simulink model "code_gen_HeadingHold"  (Simulink 7.5)
settings: Solver=FixedStepDiscrete  SolverMode=SingleTasking  StartTime=0.0  StopTime=10.0  FixedStep=0.01  RelTol=1e-3
InitFcn:
  | boat_constants
values from neighbouring files (symbols this model uses):
  figure8_waypoints = int32([ ... (first row only)    [boat_constants.m]
  OC2max = 49999    [boat_constants.m]    (also in simulation_constants.m)
  sampling_waypoints = int32([ ... (first row only)    [boat_constants.m]
  T_step = 0.01    [boat_constants.m]    (also in common.m)
  test_waypoints = int32([ ... (first row only)    [boat_constants.m]
undefined symbols (not defined in the file or in its folder): clearGpsData, clearSensorData, cpInitCommunications, DataEEInitAndClear, DataEEWrite, DiscIntNeverNeededParam, ecan1_buffered_transmit_matlab, ecan1_error_status_matlab, ecan1_init, ecan1_receive_matlab, getGpsData, getSensorData, Init_onlyOnce, Init_Reset, initCalibrationRange, initGps, processNewCommData, processNewGpsData, setHilMode, u1, u2, uart1EnqueueStateData, uart2EnqueueActuatorData, y1
libraries: simulink x85, dsPICdrivers x44, uSimLib x6, simulink_need_slupdate x4, aerolibconvert2 x2
(part 3 of 6)

== system code_gen_HeadingHold/Sensor Inputs/Change UART Baudrate ==
  HIL : Inport
  Enable : EnablePort
  Data Type Conversion : DataTypeConversion  OutDataType=fixdt(1, 16)  OutScaling=2^0
  Reconfigure UART2 baud rate [commProtocol.c] : dsPICdrivers/OTHERS/C Function Call  Tag=dsPIC_dsPIC_CFunctionCall  FctUpdate=Output Function  fctName='setHilMode'  INPUT_SIZE=1  INPUT1=uint8  INPUT2=--  INPUT3=--  OUTPUT_SIZE=1  OUTPUT1=--  SampleTime=T_step  InputType=[ 2 ]  OutputType=[ ]  FctDeclaration=extern void setHilMode(uint8_T u1);  FctCall=setHilMode(%u1);  OrderingInOutPopup=None  FctStart=None  FctStart_Name=Init_onlyOnce  FctStart_Declaration=inline extern void Init_onlyOnce();  FctStart_Call=Init_onlyOnce();  FctInit=None  FctInit_Name=Init_Reset  FctInit_Declaration=inline extern void Init_Reset();  FctInit_Call=Init_Reset();  PinDigitalInput=[]  PinDigitalOutput=[]  AnalogueInput=[]
  wires:
  HIL/1 -> Data Type Conversion/1
  Data Type Conversion/1 -> Reconfigure UART2 baud rate [commProtocol.c]/1

== system code_gen_HeadingHold/Sensor Inputs/Estop detection ==
  note: The below ECAN1 RX block is for checking for status messages.
      | If a status message hasn't been received for 2.1 seconds, a reset
      | signal is activated. The status messages for the ACS300 are not
      | sent when it is in reset, so this will catch when the estop is active.
      |
      | This also serves to check that the CAN hardware is working correctly,
      | which I have had trouble with in the past.
  Compare To Constant : simulink/Logic and Bit Operations/Compare To Constant  SystemSampleTime=-1  relop===  const=1026  LogicOutDataTypeMode=boolean
  Compare To Constant1 : simulink/Logic and Bit Operations/Compare To Constant  SystemSampleTime=-1  relop===  const=1  LogicOutDataTypeMode=boolean
  Constant1 : Constant  OutDataTypeMode=uint8  OutDataType=fixdt(1, 16)  OutScaling=2^0  OutDataTypeStr=uint8
  Data Store Memory : DataStoreMemory  DataStoreName=v_rpm  ReadBeforeWriteMsg=warning  WriteAfterWriteMsg=warning  WriteAfterReadMsg=warning  DataType=int16  OutDataType=fixdt(1, 16)  OutScaling=2^0  OutDataTypeStr=int16
  Data Store Read : DataStoreRead  Priority=2  DataStoreName=v_rpm  SampleTime=T_step
  Discrete-Time Integrator : DiscreteIntegrator  IntegratorMethod=Accumulation: Forward Euler  gainval=1  ExternalReset=level  SampleTime=-1  OutDataType=fixdt(1, 16)  OutScaling=2^0  LimitOutput=on  UpperSaturationLimit=50  LowerSaturationLimit=0  ShowSaturationPort=on  ICPrevOutput=DiscIntNeverNeededParam  ICPrevScaledInput=DiscIntNeverNeededParam
  If Action Subsystem : Subsystem  Priority=1  TreatAsAtomicUnit=on
  If1 : If  IfExpression=u1 == 1026  ShowElse=off
  Logical Operator5 : Logic  AllPortsSameDT=off  OutDataTypeMode=boolean  LogicDataType=fixdt(0, 8)  OutDataTypeStr=boolean
  Receive ECAN1 Message : Subsystem  mask(ECAN 1 Reception Block){ecan1_receive_sample_time=.01}
      mask prompts: ecan1_receive_sample_time "Sampling time"
      mask help:
      | This block will receive CAN messages over the ECAN1 peripheral on the dsPIC33f.
      | Outputs:
      | identifier - uint32 containing SID and EID
      | data - Variable-sized array (between 0 and 8) of uint8s
      | remote - boolean value specifying if this is a remote transmit request
      mask Display: disp('ECAN1 RX');
  Terminator1 : Terminator
  Terminator2 : Terminator
  Terminator3 : Terminator
  reset_estop : Outport
  tag scope: v_rpm=global
  wires:
  Receive ECAN1 Message/1(identifier) -> Compare To Constant/1, If1/1
  Constant1/1 -> Discrete-Time Integrator/1
  Compare To Constant/1 -> Logical Operator5/1
  Receive ECAN1 Message/4(new) -> Logical Operator5/2
  Logical Operator5/1 -> Discrete-Time Integrator/2
  Receive ECAN1 Message/2(data) -> If Action Subsystem/1(data)
  Receive ECAN1 Message/3(remote) -> Terminator1/1
  Receive ECAN1 Message/5(size) -> Terminator2/1
  Discrete-Time Integrator/2 -> Compare To Constant1/1
  Discrete-Time Integrator/1 -> Terminator3/1
  Compare To Constant1/1 -> reset_estop/1
  If1/1 -> If Action Subsystem/Action
  Data Store Read/1 -> [v_rpm]

== system code_gen_HeadingHold/Sensor Inputs/GPS ==
  Enable : EnablePort
  Bus Creator : BusCreator  Inputs=15
  Data Type Conversion : DataTypeConversion  OutDataTypeMode=boolean  OutDataType=fixdt(1, 16)  OutScaling=2^0  OutDataTypeStr=boolean  RndMeth=Simplest
  GPS Reception Status (LED D9) : dsPICdrivers/Digital I//O/Digital Output Write  Tag=dsPIC_Digital_Output  Priority=5  PORT=A  Pin=[6]  Simultaneous=off  OrderingInOutPopup=None
  Logical Operator4 : Logic  AllPortsSameDT=off  OutDataTypeMode=boolean  LogicDataType=fixdt(0, 8)  OutDataTypeStr=boolean
  Parse out new data since the last timestep [gps.c] : dsPICdrivers/OTHERS/C Function Call  Tag=dsPIC_dsPIC_CFunctionCall  FctUpdate=Output Function  fctName='processNewGpsData'  INPUT_SIZE=1  INPUT1=--  INPUT2=--  INPUT3=--  OUTPUT_SIZE=1  OUTPUT1=--  SampleTime=T_step  InputType=[ ]  OutputType=[ ]  FctDeclaration=extern void processNewGpsData();  FctCall=processNewGpsData();  OrderingInOutPopup=Output  FctStart=None  FctStart_Name=Init_onlyOnce  FctStart_Declaration=inline extern void Init_onlyOnce();  FctStart_Call=Init_onlyOnce();  FctInit=None  FctInit_Name=Init_Reset  FctInit_Declaration=inline extern void Init_Reset();  FctInit_Call=Init_Reset();  PinDigitalInput=[]  PinDigitalOutput=[]  AnalogueInput=[]
  Retrieve last GPS data [gps.c] : dsPICdrivers/OTHERS/C Function Call  Tag=dsPIC_dsPIC_CFunctionCall  FctUpdate=Output Function  fctName='getGpsData'  INPUT_SIZE=1  INPUT1=--  INPUT2=--  INPUT3=--  OUTPUT_SIZE=33  OUTPUT1=uint8  SampleTime=T_step  InputType=[ ]  OutputType=[ 2 ]  FctDeclaration=extern void getGpsData(uint8_T* y1);  FctCall=getGpsData(*%y1);  OrderingInOutPopup=Input  FctStart=None  FctStart_Name=Init_onlyOnce  FctStart_Declaration=inline extern void Init_onlyOnce();  FctStart_Call=Init_onlyOnce();  FctInit=None  FctInit_Name=Init_Reset  FctInit_Declaration=inline extern void Init_Reset();  FctInit_Call=Init_Reset();  PinDigitalInput=[]  PinDigitalOutput=[]  AnalogueInput=[]
  Unpack sensor data : Stateflow chart  TreatAsAtomicUnit=on
  GPS : Outport
  wires:
  Bus Creator/1 -> GPS/1
  Parse out new data since the last timestep [gps.c]/1 -> Retrieve last GPS data [gps.c]/1
  Data Type Conversion/1 -> Bus Creator/15, Logical Operator4/2  "newData"
  Unpack sensor data/15(newGpsData) -> Data Type Conversion/1
  Unpack sensor data/4(year) -> Bus Creator/4  "year"
  Unpack sensor data/5(month) -> Bus Creator/5  "month"
  Unpack sensor data/6(day) -> Bus Creator/6  "day"
  Unpack sensor data/7(hour) -> Bus Creator/7  "hour"
  Unpack sensor data/8(minute) -> Bus Creator/8  "minute"
  Unpack sensor data/9(second) -> Bus Creator/9  "second"
  Unpack sensor data/10(cog) -> Bus Creator/10  "cog"
  Unpack sensor data/11(sog) -> Bus Creator/11  "sog"
  Unpack sensor data/12(hdop) -> Bus Creator/12  "hdop"
  Unpack sensor data/13(fix) -> Bus Creator/13  "fix"
  Unpack sensor data/14(satellites) -> Bus Creator/14, Logical Operator4/1  "satellites"
  Retrieve last GPS data [gps.c]/1 -> Unpack sensor data/1(u)
  Unpack sensor data/1(latitude) -> Bus Creator/1  "latitude"
  Unpack sensor data/2(longitude) -> Bus Creator/2  "longitude"
  Unpack sensor data/3(altitude) -> Bus Creator/3  "altitude"
  Logical Operator4/1 -> GPS Reception Status (LED D9)/1

== system code_gen_HeadingHold/Sensor Inputs/Hold in reset on init ==
  note: This block outputs a 1 while it hasn't received 100 new and valid GPS fixes.
      | This counter gets reset on every transition to/from HIL mode.
  GPS : Inport
  HIL Button : Inport  Port=2
  Bus Selector : BusSelector  OutputSignals=newData,fix
  Compare To Zero : simulink/Logic and Bit Operations/Compare To Zero  SystemSampleTime=-1  relop===  LogicOutDataTypeMode=boolean
  Discrete-Time Integrator : DiscreteIntegrator  ExternalReset=either  SampleTime=-1  OutDataType=fixdt(1, 16)  OutScaling=2^0  LimitOutput=on  UpperSaturationLimit=1  LowerSaturationLimit=0  ICPrevOutput=DiscIntNeverNeededParam  ICPrevScaledInput=DiscIntNeverNeededParam
  Logical Operator : Logic  AllPortsSameDT=off  OutDataTypeMode=boolean  LogicDataType=fixdt(0, 8)  OutDataTypeStr=boolean
  Out1 : Outport
  wires:
  GPS/1 -> Bus Selector/1
  Compare To Zero/1 -> Out1/1
  Discrete-Time Integrator/1 -> Compare To Zero/1
  Bus Selector/1 -> Logical Operator/1  "<newData>"
  Bus Selector/2 -> Logical Operator/2  "<fix>"
  Logical Operator/1 -> Discrete-Time Integrator/1
  HIL Button/1 -> Discrete-Time Integrator/2

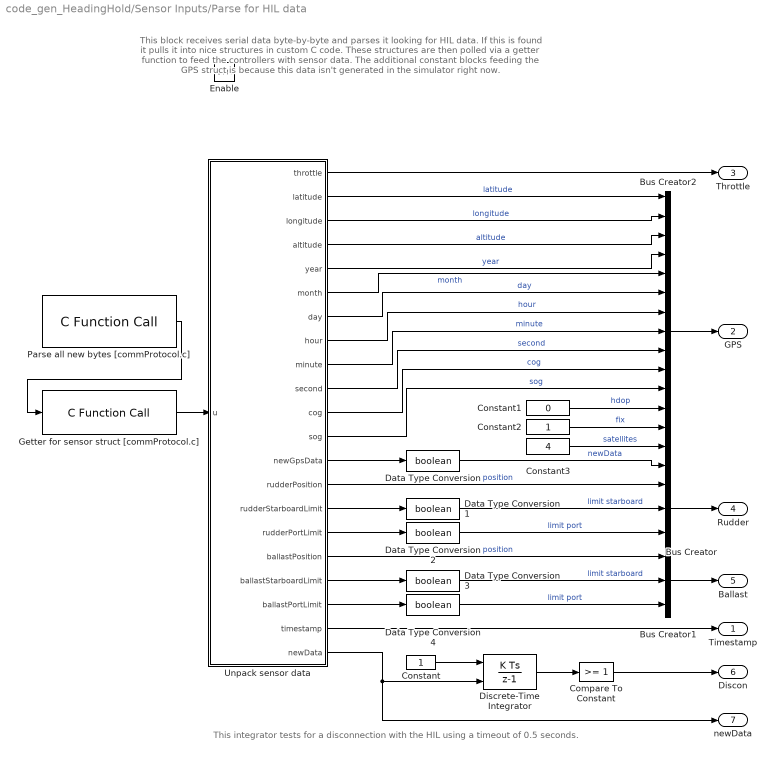
== system code_gen_HeadingHold/Sensor Inputs/Parse for HIL data ==
  note: This block receives serial data byte-by-byte and parses it looking for HIL data.
      | If this is found it pulls it into nice structures in custom C code. These structures
      | are then polled via a getter function to feed the controllers with sensor data.
      |
      | The additional constant blocks feeding the GPS struct is because this data isn't
      | generated in the simulator right now.
  note: This integrator tests for a disconnection with the HIL
      | using a timeout of 0.5 seconds.
  Enable : EnablePort
  Bus Creator : BusCreator  Inputs=3
  Bus Creator1 : BusCreator  Inputs=3
  Bus Creator2 : BusCreator  Inputs=15
  Compare To Constant : simulink/Logic and Bit Operations/Compare To Constant  SystemSampleTime=-1  relop=>=  const=1  LogicOutDataTypeMode=boolean
  Constant : Constant  OutDataTypeMode=uint8  OutDataType=fixdt(1, 16)  OutScaling=2^0  OutDataTypeStr=uint8
  Constant1 : Constant  Value=0  OutDataTypeMode=single  OutDataType=fixdt(1, 16)  OutScaling=2^0  OutDataTypeStr=single
  Constant2 : Constant  OutDataTypeMode=uint8  OutDataType=fixdt(1, 16)  OutScaling=2^0  OutDataTypeStr=uint8
  Constant3 : Constant  Value=4  OutDataTypeMode=uint8  OutDataType=fixdt(1, 16)  OutScaling=2^0  OutDataTypeStr=uint8
  Data Type Conversion{,1..4} (5 alike) : DataTypeConversion  OutDataTypeMode=boolean  OutDataType=fixdt(1, 16)  OutScaling=2^0  OutDataTypeStr=boolean
  Discrete-Time Integrator : DiscreteIntegrator  gainval=2  ExternalReset=level  SampleTime=T_step  OutDataType=fixdt(1, 16)  OutScaling=2^0  LimitOutput=on  UpperSaturationLimit=1  LowerSaturationLimit=0  ICPrevOutput=DiscIntNeverNeededParam  ICPrevScaledInput=DiscIntNeverNeededParam
  Getter for sensor struct [commProtocol.c] : dsPICdrivers/OTHERS/C Function Call  Tag=dsPIC_dsPIC_CFunctionCall  FctUpdate=Output Function  fctName='getSensorData'  INPUT_SIZE=1  INPUT1=--  INPUT2=--  INPUT3=--  OUTPUT_SIZE=40  OUTPUT1=uint8  SampleTime=.01  InputType=[ ]  OutputType=[ 2 ]  FctDeclaration=extern void getSensorData(uint8_T* y1);  FctCall=getSensorData(*%y1);  OrderingInOutPopup=Input  FctStart=None  FctStart_Name=Init_onlyOnce  FctStart_Declaration=inline extern void Init_onlyOnce();  FctStart_Call=Init_onlyOnce();  FctInit=None  FctInit_Name=Init_Reset  FctInit_Declaration=inline extern void Init_Reset();  FctInit_Call=Init_Reset();  PinDigitalInput=[]  PinDigitalOutput=[]  AnalogueInput=[]
  Parse all new bytes [commProtocol.c] : dsPICdrivers/OTHERS/C Function Call  Tag=dsPIC_dsPIC_CFunctionCall  FctUpdate=Output Function  fctName='processNewCommData'  INPUT_SIZE=1  INPUT1=--  INPUT2=--  INPUT3=--  OUTPUT_SIZE=1  OUTPUT1=--  SampleTime=.01  InputType=[ ]  OutputType=[ ]  FctDeclaration=extern void processNewCommData();  FctCall=processNewCommData();  OrderingInOutPopup=Output  FctStart=None  FctStart_Name=Init_onlyOnce  FctStart_Declaration=inline extern void Init_onlyOnce();  FctStart_Call=Init_onlyOnce();  FctInit=None  FctInit_Name=Init_Reset  FctInit_Declaration=inline extern void Init_Reset();  FctInit_Call=Init_Reset();  PinDigitalInput=[]  PinDigitalOutput=[]  AnalogueInput=[]
  Unpack sensor data : Stateflow chart  TreatAsAtomicUnit=on
  Timestamp : Outport
  GPS : Outport  Port=2
  Throttle : Outport  Port=3
  Rudder : Outport  Port=4
  Ballast : Outport  Port=5
  Discon : Outport  Port=6
  newData : Outport  Port=7
  wires:
  Unpack sensor data/1(throttle) -> Throttle/1
  Bus Creator/1 -> Rudder/1
  Bus Creator1/1 -> Ballast/1
  Bus Creator2/1 -> GPS/1
  Unpack sensor data/4(altitude) -> Bus Creator2/3  "altitude"
  Unpack sensor data/3(longitude) -> Bus Creator2/2  "longitude"
  Unpack sensor data/2(latitude) -> Bus Creator2/1  "latitude"
  Unpack sensor data/10(second) -> Bus Creator2/9  "second"
  Unpack sensor data/9(minute) -> Bus Creator2/8  "minute"
  Unpack sensor data/8(hour) -> Bus Creator2/7  "hour"
  Unpack sensor data/7(day) -> Bus Creator2/6  "day"
  Unpack sensor data/6(month) -> Bus Creator2/5  "month"
  Unpack sensor data/5(year) -> Bus Creator2/4  "year"
  Unpack sensor data/11(cog) -> Bus Creator2/10  "cog"
  Unpack sensor data/12(sog) -> Bus Creator2/11  "sog"
  Getter for sensor struct [commProtocol.c]/1 -> Unpack sensor data/1(u)
  Parse all new bytes [commProtocol.c]/1 -> Getter for sensor struct [commProtocol.c]/1
  Unpack sensor data/13(newGpsData) -> Data Type Conversion/1
  Unpack sensor data/14(rudderPosition) -> Bus Creator/1  "position"
  Unpack sensor data/15(rudderStarboardLimit) -> Data Type Conversion1/1
  Unpack sensor data/16(rudderPortLimit) -> Data Type Conversion2/1
  Unpack sensor data/17(ballastPosition) -> Bus Creator1/1  "position"
  Unpack sensor data/18(ballastStarboardLimit) -> Data Type Conversion3/1
  Unpack sensor data/19(ballastPortLimit) -> Data Type Conversion4/1
  Unpack sensor data/20(timestamp) -> Timestamp/1
  Constant/1 -> Discrete-Time Integrator/1
  Discrete-Time Integrator/1 -> Compare To Constant/1
  Unpack sensor data/21(newData) -> Discrete-Time Integrator/2, newData/1
  Compare To Constant/1 -> Discon/1
  Constant1/1 -> Bus Creator2/12  "hdop"
  Constant2/1 -> Bus Creator2/13  "fix"
  Constant3/1 -> Bus Creator2/14  "satellites"
  Data Type Conversion/1 -> Bus Creator2/15  "newData"
  Data Type Conversion1/1 -> Bus Creator/2  "limit starboard"
  Data Type Conversion2/1 -> Bus Creator/3  "limit port"
  Data Type Conversion3/1 -> Bus Creator1/2  "limit starboard"
  Data Type Conversion4/1 -> Bus Creator1/3  "limit port"

== system code_gen_HeadingHold/Sensor Inputs/Rudder Sensors ==
  note: The rudder has two main sensors: hall effect and a potentiometer. The
      | potentiometer returns a voltage value through the onboard ADC indicating
      | rudder position exactly. The three Hall effect sensors are used as limit switches
      | indicating port and starboard limits as well as center, though this sensor isn't
      | being used currently.
      |
      | It expects a range of 1.12-2.11V for the rudder position potentiometer with
      | 2.11V being hard to port. The potentiometer was powered at 3.3V for these
      | measurements.
  ADC in : Inport  OutDataType=fixdt(1, 16)  OutScaling=2^0
  Bus Creator : BusCreator  Inputs=3
  Logical Operator : Logic  Operator=NOT  Inputs=1  AllPortsSameDT=off  OutDataTypeMode=boolean  LogicDataType=fixdt(0, 8)  OutDataTypeStr=boolean
  Logical Operator1 : Logic  Operator=NOT  Inputs=1  AllPortsSameDT=off  OutDataTypeMode=boolean  LogicDataType=fixdt(0, 8)  OutDataTypeStr=boolean
  Port Hall : dsPICdrivers/Digital I//O/Digital Input  Tag=dsPIC_Digital_Input  PORT=C  Pin=[2]  SampleTime=.01  OrderingInOutPopup=None
  Starboard Hall : dsPICdrivers/Digital I//O/Digital Input  Tag=dsPIC_Digital_Input  PORT=G  Pin=[3]  SampleTime=.01  OrderingInOutPopup=None
  Weighted Moving Average : simulink_need_slupdate/Weighted Moving Average  mgainval=[.25 .25 .25 .25]  vinit=0.0  samptime=-1  OutDataTypeStr=Inherit: Inherit via back propagation  OutDataType=sfix(16)  OutScaling=2^-10  DoSatur=off  GainDataType=uint(16)  MatRadixGroup=Best Precision: Matrix-wise  GainScaling=2^-10
  Out1 : Outport
  wires:
  ADC in/1 -> Weighted Moving Average/1
  Starboard Hall/1 -> Logical Operator1/1
  Port Hall/1 -> Logical Operator/1
  Bus Creator/1 -> Out1/1
  Logical Operator/1 -> Bus Creator/3  "limit port"
  Logical Operator1/1 -> Bus Creator/2  "limit starboard"
  Weighted Moving Average/1 -> Bus Creator/1  "position"

== system code_gen_HeadingHold/Sensor Inputs/Throttle Sensors ==
  note: Throttle output is currently being ignored. The motor driver board
      | should report current velocity along with other status information
      | on a regular basis and that could be parsed for this information. As
      | of right now it's been deemed non-critical and therefore ignored.
  Constant : Constant  Value=0  OutDataTypeMode=int16  OutDataType=fixdt(1, 16)  OutScaling=2^0  OutDataTypeStr=int16  SampleTime=.01
  Out1 : Outport
  wires:
  Constant/1 -> Out1/1

== system code_gen_HeadingHold/Transmit actuator data/Package and Transmit Sensor Struct ==
  command_r : Inport
  command_b : Inport  Port=2
  command_t : Inport  Port=3
  timstamp : Inport  Port=4
  rudderAngle : Inport  Port=5
  sensorOverride : Inport  Port=6
  Enable : EnablePort
  Add actuator commands to transmission FIFO [commProtocol.c] : dsPICdrivers/OTHERS/C Function Call  Tag=dsPIC_dsPIC_CFunctionCall  FctUpdate=Output Function  fctName='uart2EnqueueActuatorData'  INPUT_SIZE=34  INPUT1=uint8  INPUT2=--  INPUT3=--  OUTPUT_SIZE=1  OUTPUT1=--  SampleTime=-1  InputType=[ 2 ]  OutputType=[ ]  FctDeclaration=extern void uart2EnqueueActuatorData(uint8_T* u1);  FctCall=uart2EnqueueActuatorData(*%u1);  OrderingInOutPopup=None  FctStart=None  FctStart_Name=Init_onlyOnce  FctStart_Declaration=inline extern void Init_onlyOnce();  FctStart_Call=Init_onlyOnce();  FctInit=None  FctInit_Name=Init_Reset  FctInit_Declaration=inline extern void Init_Reset();  FctInit_Call=Init_Reset();  PinDigitalInput=[]  PinDigitalOutput=[]  AnalogueInput=[]
  Build HIL sentence : Subsystem
  Bus Selector : BusSelector  OutputSignals=enable,direction,up,period
  Bus Selector1 : BusSelector  OutputSignals=identifier,data,size,trigger
  Bus Selector2 : BusSelector  OutputSignals=enable,direction
  Pack : Stateflow chart  TreatAsAtomicUnit=on
  wires:
  Bus Selector/2 -> Pack/2(r_dir)  "<direction>"
  Bus Selector/1 -> Pack/1(r_en)  "<enable>"
  Bus Selector1/4 -> Pack/10(t_trig)  "<trigger>"
  Bus Selector1/1 -> Pack/7(t_id)  "<identifier>"
  Bus Selector/3 -> Pack/3(r_up)  "<up>"
  Bus Selector2/1 -> Pack/5(b_en)  "<enable>"
  Bus Selector2/2 -> Pack/6(b_dir)  "<direction>"
  Bus Selector/4 -> Pack/4(r_per)  "<period>"
  Bus Selector1/2 -> Pack/8(t_data)  "<data>"
  Bus Selector1/3 -> Pack/9(t_size)  "<size>"
  command_r/1 -> Bus Selector/1
  command_b/1 -> Bus Selector2/1
  command_t/1 -> Bus Selector1/1
  timstamp/1 -> Pack/11(time)
  Build HIL sentence/1(sent) -> Add actuator commands to transmission FIFO [commProtocol.c]/1
  Pack/1(y) -> Build HIL sentence/1(data)
  rudderAngle/1 -> Pack/12(rudderAngle)
  sensorOverride/1 -> Pack/13(sensorOverride)

== system code_gen_HeadingHold/Transmit state data via UART1/Build HIL sentence ==
  data : Inport
  Bitwise Operator : simulink/Logic and Bit Operations/Bitwise Operator  logicop=XOR  UseBitMask=off  BitMask=bin2dec('11011001')  BitMaskRealWorld=Stored Integer
  Constant : Constant  Value=37  OutDataTypeMode=uint8  OutDataType=fixdt(1, 16)  OutScaling=2^0  OutDataTypeStr=uint8
  Constant1 : Constant  Value=38  OutDataTypeMode=uint8  OutDataType=fixdt(1, 16)  OutScaling=2^0  OutDataTypeStr=uint8
  Constant2 : Constant  Value=94  OutDataTypeMode=uint8  OutDataType=fixdt(1, 16)  OutScaling=2^0  OutDataTypeStr=uint8
  Constant3 : Constant  Value=38  OutDataTypeMode=uint8  OutDataType=fixdt(1, 16)  OutScaling=2^0  OutDataTypeStr=uint8
  Constant4 : Constant  Value=3  OutDataTypeMode=uint8  OutDataType=fixdt(1, 16)  OutScaling=2^0  OutDataTypeStr=uint8
  Mux2 : Mux  Inputs=3
  Pack : Stateflow chart  TreatAsAtomicUnit=on
  Probe : Probe  ProbeSampleTime=off  ProbeComplexSignal=off  ProbeWidthDataType=uint8
  sent : Outport
  wires:
  data/1 -> Probe/1, Mux2/3
  Constant/1 -> Pack/1(a)
  Constant1/1 -> Pack/2(b)
  Pack/1(y) -> sent/1
  Mux2/1 -> Bitwise Operator/1, Pack/3(c)
  Probe/1 -> Mux2/2
  Constant2/1 -> Pack/4(d)
  Constant3/1 -> Pack/5(e)
  Bitwise Operator/1 -> Pack/6(f)
  Constant4/1 -> Mux2/1

== system code_gen_HeadingHold/Actuator Outputs/To Drive Motor/C-function Call ==
  parameters : Inport  OutDataType=sfix(16)  OutScaling=2^0
  Enable : EnablePort
  ECAN1 Transmit [ecanFunctions.c] : dsPICdrivers/OTHERS/C Function Call  Tag=dsPIC_dsPIC_CFunctionCall  FctUpdate=Output Function  fctName='ecan1_buffered_transmit_matlab'  INPUT_SIZE=8  INPUT1=uint16  INPUT2=--  INPUT3=--  OUTPUT_SIZE=1  OUTPUT1=--  SampleTime=c_func_sample_time  InputType=[ 4 ]  OutputType=[ ]  FctDeclaration=extern void ecan1_buffered_transmit_matlab(uint16_T* u1);  FctCall=ecan1_buffered_transmit_matlab(*%u1);  OrderingInOutPopup=None  FctStart=None  FctStart_Name=Init_onlyOnce  FctStart_Declaration=inline extern void Init_onlyOnce();  FctStart_Call=Init_onlyOnce();  FctInit=None  FctInit_Name=Init_Reset  FctInit_Declaration=inline extern void Init_Reset();  FctInit_Call=Init_Reset();  PinDigitalInput=[]  PinDigitalOutput=[]  AnalogueInput=[]
  wires:
  parameters/1 -> ECAN1 Transmit [ecanFunctions.c]/1

== system code_gen_HeadingHold/Actuator Outputs/To Drive Motor/uint8 combiner1 ==
  high-order : Inport  OutDataType=sfix(16)  OutScaling=2^0
  low-order : Inport  Port=2  OutDataType=sfix(16)  OutScaling=2^0
  Bitwise Operator : simulink/Logic and Bit Operations/Bitwise Operator  logicop=OR  UseBitMask=off  NumInputPorts=2  BitMask=bin2dec('11011001')  BitMaskRealWorld=Stored Integer
  Data Type Conversion : DataTypeConversion  OutDataTypeMode=uint16  OutDataType=sfix(16)  OutScaling=2^0  OutDataTypeStr=uint16
  Data Type Conversion1 : DataTypeConversion  OutDataTypeMode=uint16  OutDataType=sfix(16)  OutScaling=2^0  OutDataTypeStr=uint16
  Shift Arithmetic : simulink/Logic and Bit Operations/Shift Arithmetic  SystemSampleTime=-1  nBitShiftRight=-8  nBinPtShiftRight=0
  combined : Outport  OutDataType=sfix(16)  OutScaling=2^0
  wires:
  low-order/1 -> Data Type Conversion/1
  Bitwise Operator/1 -> combined/1
  high-order/1 -> Data Type Conversion1/1
  Shift Arithmetic/1 -> Bitwise Operator/2
  Data Type Conversion/1 -> Shift Arithmetic/1
  Data Type Conversion1/1 -> Bitwise Operator/1

== system code_gen_HeadingHold/Actuator Outputs/To Drive Motor/uint8 combiner2 ==
  high-order : Inport  OutDataType=sfix(16)  OutScaling=2^0
  low-order : Inport  Port=2  OutDataType=sfix(16)  OutScaling=2^0
  Bitwise Operator : simulink/Logic and Bit Operations/Bitwise Operator  logicop=OR  UseBitMask=off  NumInputPorts=2  BitMask=bin2dec('11011001')  BitMaskRealWorld=Stored Integer
  Data Type Conversion : DataTypeConversion  OutDataTypeMode=uint16  OutDataType=sfix(16)  OutScaling=2^0  OutDataTypeStr=uint16
  Data Type Conversion1 : DataTypeConversion  OutDataTypeMode=uint16  OutDataType=sfix(16)  OutScaling=2^0  OutDataTypeStr=uint16
  Shift Arithmetic : simulink/Logic and Bit Operations/Shift Arithmetic  SystemSampleTime=-1  nBitShiftRight=-8  nBinPtShiftRight=0
  combined : Outport  OutDataType=sfix(16)  OutScaling=2^0
  wires:
  Data Type Conversion1/1 -> Bitwise Operator/1
  Data Type Conversion/1 -> Shift Arithmetic/1
  Shift Arithmetic/1 -> Bitwise Operator/2
  high-order/1 -> Data Type Conversion1/1
  Bitwise Operator/1 -> combined/1
  low-order/1 -> Data Type Conversion/1

== system code_gen_HeadingHold/Controller/Auto/Manual Switch/If Action Subsystem ==
  r_i : Inport  OutDataType=fixdt(1, 16)  OutScaling=2^0
  t_i : Inport  Port=2  OutDataType=fixdt(1, 16)  OutScaling=2^0
  Action Port : ActionPort  ActionType=else
  Signal Conversion : SignalConversion  ConversionOutput=Bus copy
  Signal Conversion1 : SignalConversion  ConversionOutput=Bus copy
  r_o : Outport  OutDataType=fixdt(1, 16)  OutScaling=2^0
  t_o : Outport  Port=2  OutDataType=fixdt(1, 16)  OutScaling=2^0
  wires:
  r_i/1 -> Signal Conversion/1
  t_i/1 -> Signal Conversion1/1
  Signal Conversion/1 -> r_o/1
  Signal Conversion1/1 -> t_o/1

== system code_gen_HeadingHold/Controller/Auto/Manual Switch/If Action Subsystem1 ==
  r_i : Inport  OutDataType=fixdt(1, 16)  OutScaling=2^0
  t_i : Inport  Port=2  OutDataType=fixdt(1, 16)  OutScaling=2^0
  Action Port : ActionPort  ActionType=then
  Signal Conversion : SignalConversion  ConversionOutput=Bus copy
  Signal Conversion1 : SignalConversion  ConversionOutput=Bus copy
  r_o : Outport  OutDataType=fixdt(1, 16)  OutScaling=2^0
  t_o : Outport  Port=2  OutDataType=fixdt(1, 16)  OutScaling=2^0
  wires:
  r_i/1 -> Signal Conversion1/1
  t_i/1 -> Signal Conversion/1
  Signal Conversion/1 -> t_o/1
  Signal Conversion1/1 -> r_o/1

== system code_gen_HeadingHold/Controller/Auto/Manual Switch/If Action Subsystem2 ==
  r_i : Inport  OutDataType=fixdt(1, 16)  OutScaling=2^0
  t_i : Inport  Port=2  OutDataType=fixdt(1, 16)  OutScaling=2^0
  Action Port : ActionPort  ActionType=else
  Signal Conversion : SignalConversion  ConversionOutput=Bus copy
  Signal Conversion1 : SignalConversion  ConversionOutput=Bus copy
  r_o : Outport  OutDataType=fixdt(1, 16)  OutScaling=2^0
  t_o : Outport  Port=2  OutDataType=fixdt(1, 16)  OutScaling=2^0
  wires:
  r_i/1 -> Signal Conversion/1
  t_i/1 -> Signal Conversion1/1
  Signal Conversion/1 -> r_o/1
  Signal Conversion1/1 -> t_o/1

== system code_gen_HeadingHold/Controller/Auto/Manual Switch/If Action Subsystem3 ==
  r_i : Inport  OutDataType=fixdt(1, 16)  OutScaling=2^0
  t_i : Inport  Port=2  OutDataType=fixdt(1, 16)  OutScaling=2^0
  Action Port : ActionPort  ActionType=then
  Signal Conversion : SignalConversion  ConversionOutput=Bus copy
  Signal Conversion1 : SignalConversion  ConversionOutput=Bus copy
  r_o : Outport  OutDataType=fixdt(1, 16)  OutScaling=2^0
  t_o : Outport  Port=2  OutDataType=fixdt(1, 16)  OutScaling=2^0
  wires:
  r_i/1 -> Signal Conversion1/1
  t_i/1 -> Signal Conversion/1
  Signal Conversion/1 -> t_o/1
  Signal Conversion1/1 -> r_o/1

== system code_gen_HeadingHold/Controller/Auto/Manual Switch/Rudder calibration controller ==
  sensors_r : Inport
  rudder_angle : Inport  Port=2
  trigger : Inport  Port=3
  Bus Selector : BusSelector  OutputSignals=limit port,limit starboard
  Rudder Command : Subsystem
  Run rudder for calibration : Stateflow chart  TreatAsAtomicUnit=on
  Throttle Command : Subsystem
  mode : Outport
  command_r : Outport  Port=2
  command_t : Outport  Port=3
  wires:
  trigger/1 -> Run rudder for calibration/1(trigger)
  Bus Selector/1 -> Run rudder for calibration/2(rudder_port_limit)  "<limit port>"
  Bus Selector/2 -> Run rudder for calibration/3(rudder_sb_limit)  "<limit starboard>"
  Run rudder for calibration/1(step) -> Rudder Command/1(step)
  Run rudder for calibration/2(dir) -> Rudder Command/2(dir)
  Run rudder for calibration/3(throttle) -> Throttle Command/1(en)
  sensors_r/1 -> Bus Selector/1
  rudder_angle/1 -> Run rudder for calibration/4(rudder_position)
  Throttle Command/1(command) -> command_t/1
  Rudder Command/1(Command) -> command_r/1
  Run rudder for calibration/4(mode) -> mode/1

== system code_gen_HeadingHold/Controller/Autonomous Controller/Ballast Command ==
  Bus Creator : BusCreator  Inputs=2
  Constant : Constant  Value=0  OutDataTypeMode=boolean  OutDataType=fixdt(1, 16)  OutScaling=2^0  OutDataTypeStr=boolean
  Constant1 : Constant  Value=0  OutDataTypeMode=boolean  OutDataType=fixdt(1, 16)  OutScaling=2^0  OutDataTypeStr=boolean
  c_ballast : Outport
  wires:
  Constant1/1 -> Bus Creator/2  "direction"
  Constant/1 -> Bus Creator/1  "enable"
  Bus Creator/1 -> c_ballast/1

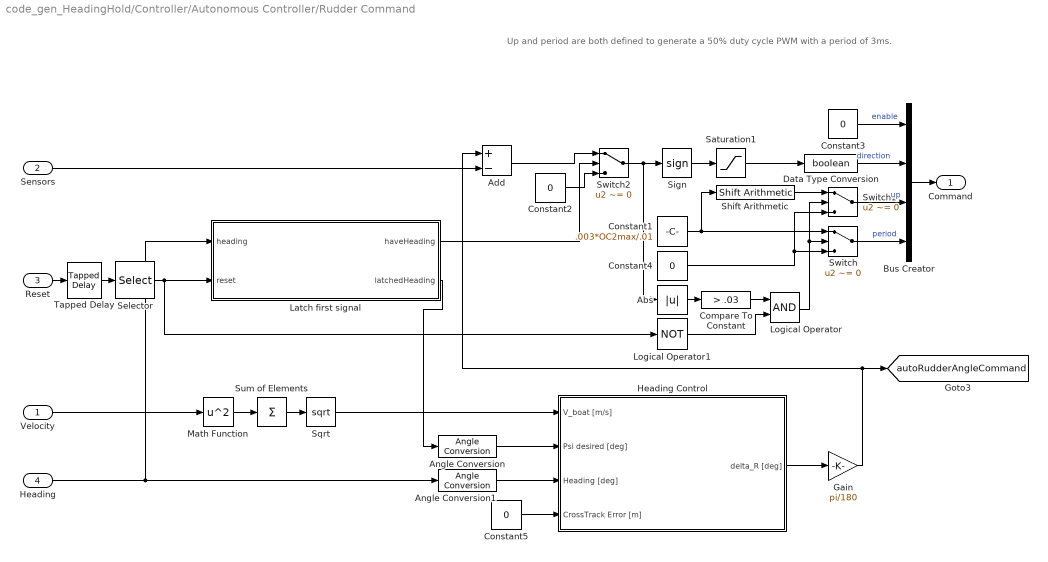
== system code_gen_HeadingHold/Controller/Autonomous Controller/Rudder Command ==
  note: Up and period are both defined to generate a 50% duty cycle PWM with
      | a period of 3ms.
  Velocity : Inport
  Sensors : Inport  Port=2
  Reset : Inport  Port=3
  Heading : Inport  Port=4
  Abs : Abs  OutDataType=fixdt(1, 16)  OutScaling=2^0
  Add : Sum  Inputs=+-  OutDataType=fixdt(1, 16)  OutScaling=2^-10
  Angle Conversion : uSimLib/Conversions/Angle Conversion  SystemSampleTime=-1  iu=rad  ou=deg
  Angle Conversion1 : uSimLib/Conversions/Angle Conversion  SystemSampleTime=-1  iu=rad  ou=deg
  Bus Creator : BusCreator
  Compare To Constant : simulink/Logic and Bit Operations/Compare To Constant  SystemSampleTime=-1  relop=>  const=.03  LogicOutDataTypeMode=boolean
  Constant1 : Constant  Value=.003*OC2max/.01  OutDataTypeMode=uint16  OutDataType=sfix(16)  OutScaling=2^0  OutDataTypeStr=uint16
  Constant2 : Constant  Value=0  OutDataTypeMode=single  OutDataType=sfix(16)  OutScaling=2^0  OutDataTypeStr=single
  Constant3 : Constant  Value=0  OutDataTypeMode=boolean  OutDataType=sfix(16)  OutScaling=2^0  OutDataTypeStr=boolean
  Constant4 : Constant  Value=0  OutDataTypeMode=uint16  OutDataType=sfix(16)  OutScaling=2^0  OutDataTypeStr=uint16
  Constant5 : Constant  Value=0  OutDataTypeMode=uint8  OutDataType=sfix(16)  OutScaling=2^0  OutDataTypeStr=uint8
  Data Type Conversion : DataTypeConversion  OutDataTypeMode=boolean  OutDataType=fixdt(1, 16)  OutScaling=2^0  OutDataTypeStr=boolean  RndMeth=Simplest
  Gain : Gain  Gain=pi/180  ParameterDataType=fixdt(1, 16)  ParameterScaling=2^0  OutDataTypeMode=single  OutDataType=fixdt(1, 16)  OutScaling=2^0  OutDataTypeStr=single
  Heading Control : Subsystem
  Latch first signal : Stateflow chart  TreatAsAtomicUnit=on
  Logical Operator : Logic  AllPortsSameDT=off  OutDataTypeMode=boolean  LogicDataType=fixdt(0, 8)  OutDataTypeStr=boolean
  Logical Operator1 : Logic  Operator=NOT  Inputs=1  AllPortsSameDT=off  OutDataTypeMode=boolean  LogicDataType=fixdt(0, 8)  OutDataTypeStr=boolean
  Math Function : Math  Operator=square  OutDataType=fixdt(1, 16)  OutScaling=2^0  SaturateOnIntegerOverflow=on
  Saturation1 : Saturate  UpperLimit=1  LowerLimit=0  OutDataTypeStr=Inherit: Inherit via back propagation
  Selector : Selector  InputPortWidth=100  IndexOptions=Index vector (dialog)  Indices=1  OutputSizes=1
  Shift Arithmetic : simulink/Logic and Bit Operations/Shift Arithmetic  SystemSampleTime=-1  nBitShiftRight=1  nBinPtShiftRight=0
  Sign : Signum
  Sqrt : Sqrt  OutDataTypeMode=single  OutDataTypeStr=single  SaturateOnIntegerOverflow=on
  Sum of Elements : Sum  Inputs=+  OutDataTypeMode=single  OutDataType=fixdt(1, 16)  OutScaling=2^-10  OutDataTypeStr=single
  Switch : Switch  Criteria=u2 ~= 0  OutDataType=fixdt(1, 16)  OutScaling=2^0
  Switch1 : Switch  Criteria=u2 ~= 0  OutDataType=fixdt(1, 16)  OutScaling=2^0
  Switch2 : Switch  Criteria=u2 ~= 0  OutDataType=fixdt(1, 16)  OutScaling=2^0
  Tapped Delay : simulink/Discrete/Tapped Delay  vinit=0  samptime=-1  NumDelays=100  DelayOrder=Oldest  includeCurrent=off
  Command : Outport
  tag scope: autoRudderAngleCommand=global
  wires:
  Angle Conversion1/1 -> Heading Control/3(Heading [deg])
  Gain/1 -> Add/1, [autoRudderAngleCommand]
  Heading Control/1(delta_R [deg]) -> Gain/1
  Sum of Elements/1 -> Sqrt/1
  Math Function/1 -> Sum of Elements/1
  Sqrt/1 -> Heading Control/1(V_boat [m/s])
  Constant5/1 -> Heading Control/4(CrossTrack Error [m])
  Heading/1 -> Angle Conversion1/1, Latch first signal/1(heading)
  Logical Operator1/1 -> Logical Operator/2
  Logical Operator/1 -> Switch1/2, Switch/2
  Compare To Constant/1 -> Logical Operator/1
  Reset/1 -> Tapped Delay/1
  Constant4/1 -> Switch1/3, Switch/3
  Switch1/1 -> Bus Creator/3  "up"
  Switch/1 -> Bus Creator/4  "period"
  Shift Arithmetic/1 -> Switch1/1
  Abs/1 -> Compare To Constant/1
  Constant1/1 -> Switch/1, Shift Arithmetic/1
  Constant3/1 -> Bus Creator/1  "enable"
  Velocity/1 -> Math Function/1
  Sign/1 -> Saturation1/1
  Saturation1/1 -> Data Type Conversion/1
  Bus Creator/1 -> Command/1
  Sensors/1 -> Add/2
  Data Type Conversion/1 -> Bus Creator/2  "direction"
  Latch first signal/2(latchedHeading) -> Angle Conversion/1
  Latch first signal/1(haveHeading) -> Switch2/2
  Add/1 -> Switch2/1
  Constant2/1 -> Switch2/3
  Switch2/1 -> Sign/1, Abs/1
  Angle Conversion/1 -> Heading Control/2(Psi desired [deg])
  Tapped Delay/1 -> Selector/1
  Selector/1 -> Logical Operator1/1, Latch first signal/2(reset)

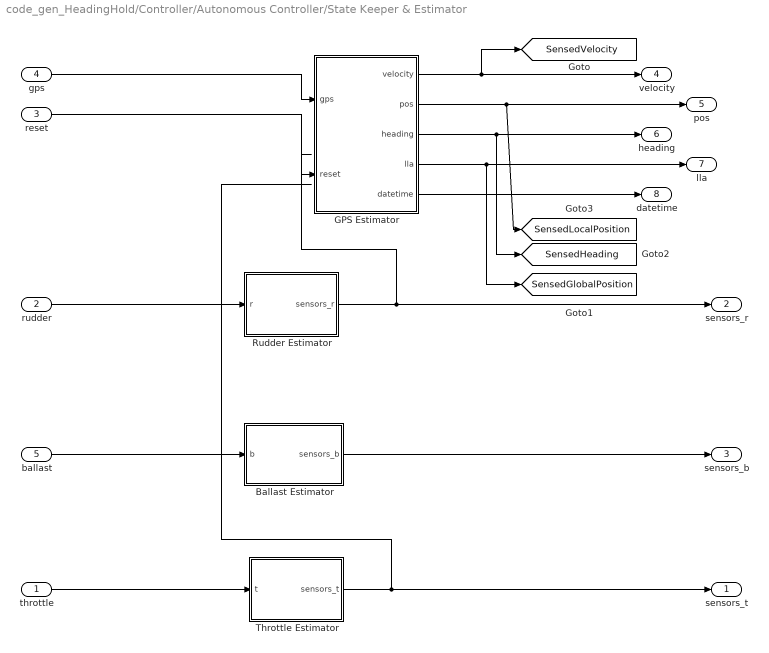
== system code_gen_HeadingHold/Controller/Autonomous Controller/State Keeper & Estimator ==
  throttle : Inport
  rudder : Inport  Port=2
  reset : Inport  Port=3
  gps : Inport  Port=4
  ballast : Inport  Port=5
  Ballast Estimator : Subsystem
  GPS Estimator : Subsystem
  Rudder Estimator : Subsystem
  Throttle Estimator : Subsystem
  sensors_t : Outport
  sensors_r : Outport  Port=2
  sensors_b : Outport  Port=3
  velocity : Outport  Port=4
  pos : Outport  Port=5
  heading : Outport  Port=6
  lla : Outport  Port=7
  datetime : Outport  Port=8
  tag scope: SensedGlobalPosition=global, SensedHeading=global, SensedLocalPosition=global, SensedVelocity=global
  wires:
  Throttle Estimator/1(sensors_t) -> sensors_t/1
  Ballast Estimator/1(sensors_b) -> sensors_b/1
  Rudder Estimator/1(sensors_r) -> sensors_r/1
  GPS Estimator/5(datetime) -> datetime/1
  GPS Estimator/4(lla) -> lla/1, [SensedGlobalPosition]
  GPS Estimator/3(heading) -> [SensedHeading], heading/1
  GPS Estimator/2(pos) -> [SensedLocalPosition], pos/1
  gps/1 -> GPS Estimator/1(gps)
  GPS Estimator/1(velocity) -> [SensedVelocity], velocity/1
  reset/1 -> GPS Estimator/2(reset)
  throttle/1 -> Throttle Estimator/1(t)
  ballast/1 -> Ballast Estimator/1(b)
  rudder/1 -> Rudder Estimator/1(r)

== system code_gen_HeadingHold/Controller/Autonomous Controller/Throttle Command ==
  sensors : Inport
  reset : Inport  Port=2
  Bus Creator : BusCreator
  Constant1 : Constant  Value=0  OutDataTypeMode=int16  OutDataType=sfix(16)  OutScaling=2^0  OutDataTypeStr=int16
  Constant5 : Constant  Value=1000  OutDataTypeMode=int16  OutDataType=sfix(16)  OutScaling=2^0  OutDataTypeStr=int16
  Mux Everything : Subsystem
  Switch : Switch  Criteria=u2 > Threshold  OutDataType=fixdt(1, 16)  OutScaling=2^0
  Terminator : Terminator
  Trigger Events : Subsystem
  command : Outport  OutDataType=sfix(16)  OutScaling=2^0
  tag scope: autoThrottleCommand=global
  wires:
  Constant5/1 -> Switch/3
  Constant1/1 -> Switch/1
  Switch/1 -> Trigger Events/1(RC Throttle), Mux Everything/4(Throttle), [autoThrottleCommand]
  Mux Everything/4(trig) -> Bus Creator/4  "trigger"
  Mux Everything/3(size) -> Bus Creator/3  "size"
  Mux Everything/2(data) -> Bus Creator/2  "data"
  Mux Everything/1(iden) -> Bus Creator/1  "identifier"
  reset/1 -> Switch/2, Trigger Events/2(Reset)
  Trigger Events/2(Disable) -> Mux Everything/2(disable)
  Trigger Events/3(Enable) -> Mux Everything/3(enable)
  Trigger Events/1(Change Speed) -> Mux Everything/1(speed)
  Bus Creator/1 -> command/1
  sensors/1 -> Terminator/1

== system code_gen_HeadingHold/Controller/RC Inputs/Map PWM values to Actuator Signals ==
  In1 : Inport
  In2 : Inport  Port=2
  rAngle : Inport  Port=3
  Enable : EnablePort
  Manual Rudder Command : Subsystem
  Throttle Command : Subsystem
  Out1 : Outport
  Out2 : Outport  Port=2
  wires:
  In1/1 -> Manual Rudder Command/1(RC Rudder)
  Manual Rudder Command/1(Rudder Command) -> Out1/1
  In2/1 -> Throttle Command/1(speed)
  Throttle Command/1(command) -> Out2/1
  rAngle/1 -> Manual Rudder Command/2(rudderAngle)

== system code_gen_HeadingHold/Controller/Radio Control Inputs1/Calibration ==
  r : Inport  OutDataType=fixdt(1, 16)  OutScaling=2^0
  tr : Inport  Port=2  OutDataType=fixdt(1, 16)  OutScaling=2^0
  t : Inport  Port=3  OutDataType=fixdt(1, 16)  OutScaling=2^0
  Enable : EnablePort
  Data Store Read : DataStoreRead  DataStoreName=throttleRange  SampleTime=T_step
  Data Store Read1 : DataStoreRead  DataStoreName=rudderRange  SampleTime=T_step
  Data Store Read2 : DataStoreRead  DataStoreName=trackRange  SampleTime=T_step
  Data Store Write : DataStoreWrite  DataStoreName=throttleRange  SampleTime=-1
  Data Store Write1 : DataStoreWrite  DataStoreName=rudderRange  SampleTime=-1
  Data Store Write2 : DataStoreWrite  DataStoreName=trackRange  SampleTime=-1
  Data Type Conversion : DataTypeConversion  OutDataTypeMode=uint16  OutDataType=fixdt(1, 16)  OutScaling=2^0  OutDataTypeStr=uint16
  Data Type Conversion1 : DataTypeConversion  OutDataTypeMode=uint16  OutDataType=fixdt(1, 16)  OutScaling=2^0  OutDataTypeStr=uint16
  Data Type Conversion2 : DataTypeConversion  OutDataTypeMode=uint16  OutDataType=fixdt(1, 16)  OutScaling=2^0  OutDataTypeStr=uint16
  Store rudder range to memory : Subsystem
  Store throttle range to memory : Subsystem
  Store track range to memory : Subsystem
  Update range from input : Subsystem
  Update range from input1 : Subsystem
  Update range from input2 : Subsystem
  wires:
  Update range from input/1(newRange) -> Data Store Write1/1, Data Type Conversion/1
  Data Store Read1/1 -> Update range from input/1(limitRange)
  r/1 -> Update range from input/2(newValue)
  Update range from input2/1(newRange) -> Data Store Write2/1, Data Type Conversion2/1
  Data Store Read2/1 -> Update range from input2/1(limitRange)
  tr/1 -> Update range from input2/2(newValue)
  Update range from input1/1(newRange) -> Data Store Write/1, Data Type Conversion1/1
  Data Store Read/1 -> Update range from input1/1(limitRange)
  t/1 -> Update range from input1/2(newValue)
  Data Type Conversion/1 -> Store rudder range to memory/1(rudderRange)
  Data Type Conversion1/1 -> Store throttle range to memory/1(throttleRange)
  Data Type Conversion2/1 -> Store track range to memory/1(trackRange)

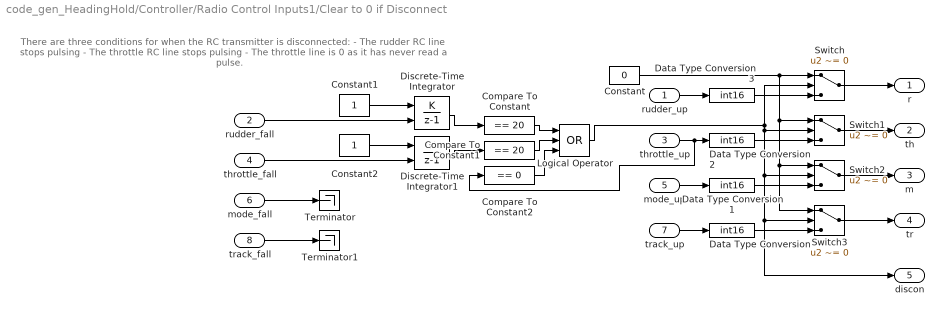
== system code_gen_HeadingHold/Controller/Radio Control Inputs1/Clear to 0 if Disconnect ==
  note: There are three conditions for when the RC transmitter is disconnected:
      |  - The rudder RC line stops pulsing
      |  - The throttle RC line stops pulsing
      |  - The throttle line is 0 as it has never read a pulse.
  rudder_up : Inport  OutDataType=sfix(16)  OutScaling=2^0
  rudder_fall : Inport  Port=2  OutDataType=sfix(16)  OutScaling=2^0
  throttle_up : Inport  Port=3  OutDataType=sfix(16)  OutScaling=2^0
  throttle_fall : Inport  Port=4  OutDataType=sfix(16)  OutScaling=2^0
  mode_up : Inport  Port=5  OutDataType=sfix(16)  OutScaling=2^0
  mode_fall : Inport  Port=6  OutDataType=sfix(16)  OutScaling=2^0
  track_up : Inport  Port=7  OutDataType=sfix(16)  OutScaling=2^0
  track_fall : Inport  Port=8  OutDataType=sfix(16)  OutScaling=2^0
  Compare To Constant : simulink/Logic and Bit Operations/Compare To Constant  SystemSampleTime=-1  relop===  const=20  LogicOutDataTypeMode=boolean
  Compare To Constant1 : simulink/Logic and Bit Operations/Compare To Constant  SystemSampleTime=-1  relop===  const=20  LogicOutDataTypeMode=boolean
  Compare To Constant2 : simulink/Logic and Bit Operations/Compare To Constant  SystemSampleTime=-1  relop===  const=0  LogicOutDataTypeMode=boolean
  Constant : Constant  Value=0  OutDataTypeMode=int16  OutDataType=sfix(16)  OutScaling=2^0  OutDataTypeStr=int16
  Constant1 : Constant  OutDataTypeMode=uint8  OutDataType=fixdt(1, 16)  OutScaling=2^0  OutDataTypeStr=uint8
  Constant2 : Constant  OutDataTypeMode=uint8  OutDataType=fixdt(1, 16)  OutScaling=2^0  OutDataTypeStr=uint8
  Data Type Conversion{,1..3} (4 alike) : DataTypeConversion  OutDataTypeMode=int16  OutDataType=fixdt(1, 16)  OutScaling=2^0  OutDataTypeStr=int16
  Discrete-Time Integrator : DiscreteIntegrator  IntegratorMethod=Accumulation: Forward Euler  ExternalReset=level  SampleTime=-1  OutDataType=fixdt(1, 16)  OutScaling=2^0  LimitOutput=on  UpperSaturationLimit=20  LowerSaturationLimit=0  ICPrevOutput=DiscIntNeverNeededParam  ICPrevScaledInput=DiscIntNeverNeededParam
  Discrete-Time Integrator1 : DiscreteIntegrator  IntegratorMethod=Accumulation: Forward Euler  ExternalReset=level  SampleTime=-1  OutDataType=fixdt(1, 16)  OutScaling=2^0  LimitOutput=on  UpperSaturationLimit=20  LowerSaturationLimit=0  ICPrevOutput=DiscIntNeverNeededParam  ICPrevScaledInput=DiscIntNeverNeededParam
  Logical Operator : Logic  Operator=OR  Inputs=3  AllPortsSameDT=off  OutDataTypeMode=boolean  LogicDataType=fixdt(0, 8)  OutDataTypeStr=boolean
  Switch{,1..3} (4 alike) : Switch  Criteria=u2 ~= 0  Threshold=40
  Terminator : Terminator
  Terminator1 : Terminator
  r : Outport  OutDataType=sfix(16)  OutScaling=2^0
  th : Outport  Port=2  OutDataType=sfix(16)  OutScaling=2^0
  m : Outport  Port=3  OutDataType=sfix(16)  OutScaling=2^0
  tr : Outport  Port=4  OutDataType=sfix(16)  OutScaling=2^0
  discon : Outport  Port=5  OutDataType=sfix(16)  OutScaling=2^0
  wires:
  Switch1/1 -> th/1
  throttle_up/1 -> Data Type Conversion2/1, Compare To Constant2/1
  Switch/1 -> r/1
  rudder_up/1 -> Data Type Conversion3/1
  Constant/1 -> Switch/1, Switch1/1, Switch2/1, Switch3/1
  Switch2/1 -> m/1
  mode_up/1 -> Data Type Conversion1/1
  track_up/1 -> Data Type Conversion/1
  Switch3/1 -> tr/1
  rudder_fall/1 -> Discrete-Time Integrator/2
  mode_fall/1 -> Terminator/1
  track_fall/1 -> Terminator1/1
  Constant1/1 -> Discrete-Time Integrator/1
  throttle_fall/1 -> Discrete-Time Integrator1/2
  Data Type Conversion/1 -> Switch3/3
  Data Type Conversion1/1 -> Switch2/3
  Data Type Conversion2/1 -> Switch1/3
  Data Type Conversion3/1 -> Switch/3
  Constant2/1 -> Discrete-Time Integrator1/1
  Logical Operator/1 -> Switch/2, Switch1/2, Switch2/2, Switch3/2, discon/1
  Discrete-Time Integrator1/1 -> Compare To Constant1/1
  Discrete-Time Integrator/1 -> Compare To Constant/1
  Compare To Constant/1 -> Logical Operator/1
  Compare To Constant1/1 -> Logical Operator/2
  Compare To Constant2/1 -> Logical Operator/3

== system code_gen_HeadingHold/Controller/Radio Control Inputs1/Detect calibration trigger ==
  note: This part checks for a mode change and checks that
      | it isn't the result of a disconnect. We don't want those
      | to accidently trigger a calibration.
  mode : Inport
  value : Inport  Port=2
  Calibration mode (LED D6) : dsPICdrivers/Digital I//O/Digital Output Write  Tag=dsPIC_Digital_Output  Priority=5  PORT=A  Pin=3  Simultaneous=off  OrderingInOutPopup=None
  Compare To Constant1 : simulink/Logic and Bit Operations/Compare To Constant  SystemSampleTime=-1  relop=>  const=0  LogicOutDataTypeMode=uint8
  Compute Calibration State : Stateflow chart  TreatAsAtomicUnit=on
  Data Store Memory : DataStoreMemory  DataStoreName=restoredCalibration  ReadBeforeWriteMsg=warning  WriteAfterWriteMsg=warning  WriteAfterReadMsg=warning  DataType=boolean  OutDataType=fixdt(1, 16)  OutScaling=2^0  OutDataTypeStr=boolean
      settings: RTWStateStorageClass=ExportedGlobal
  Data Store Read1 : DataStoreRead  DataStoreName=restoredCalibration  SampleTime=T_step
  Detect Change1 : simulink/Logic and Bit Operations/Detect Change  SystemSampleTime=-1  vinit=0
  Logical Operator : Logic  AllPortsSameDT=off  OutDataTypeMode=boolean  LogicDataType=fixdt(0, 8)  OutDataTypeStr=boolean
  State outputs : Subsystem
  calibrateState : Outport  OutDataType=fixdt(1, 16)  OutScaling=2^0
  wires:
  mode/1 -> Detect Change1/1
  Logical Operator/1 -> Compute Calibration State/1(trigger)
  State outputs/1(LED) -> Calibration mode (LED D6)/1
  value/1 -> Compare To Constant1/1
  Detect Change1/1 -> Logical Operator/1
  Compare To Constant1/1 -> Logical Operator/2
  Compute Calibration State/1(state) -> calibrateState/1, State outputs/1(cState)
  Data Store Read1/1 -> Compute Calibration State/2(restoredCalibration)

== system code_gen_HeadingHold/Controller/Radio Control Inputs1/If Action Subsystem ==
  Action Port : ActionPort  ActionType=then
  Constant : Constant  Value=0  OutDataTypeMode=single  OutDataType=fixdt(1, 16)  OutScaling=2^0  OutDataTypeStr=single
  Out1 : Outport  OutDataType=fixdt(1, 16)  OutScaling=2^0  InitialOutput=50
  wires:
  Constant/1 -> Out1/1

== system code_gen_HeadingHold/Controller/Radio Control Inputs1/If Action Subsystem1 ==
  note: This subsystem maps the input RC range into hundreds of a degree. It
      | follows the convention where positive angles are to port and negative
      | angles are to starboard.
  input : Inport  OutDataType=fixdt(1, 16)  OutScaling=2^0
  range : Inport  Port=2  OutDataType=fixdt(1, 16)  OutScaling=2^0
  Action Port : ActionPort  ActionType=else
  Add 8% center deadband : Subsystem
  Constant : Constant  Value=-450  OutDataType=fixdt(1, 16)  OutScaling=2^0  OutDataTypeStr=Inherit: Inherit via back propagation
  Constant1 : Constant  Value=450  OutDataType=fixdt(1, 16)  OutScaling=2^0  OutDataTypeStr=Inherit: Inherit via back propagation
  Data Type Conversion : DataTypeConversion  OutDataType=fixdt(1, 16)  OutScaling=2^0
  Data Type Conversion1 : DataTypeConversion  OutDataType=fixdt(1, 16)  OutScaling=2^0
  Data Type Conversion2 : DataTypeConversion  OutDataTypeMode=single  OutDataType=fixdt(1, 16)  OutScaling=2^0  OutDataTypeStr=single
  Demux : Demux  Outputs=2
  Gain : Gain  Gain=pi/1800  ParameterDataType=fixdt(1, 16)  ParameterScaling=2^0  OutDataType=fixdt(1, 16)  OutScaling=2^0
  Map into range : Stateflow chart  TreatAsAtomicUnit=on
  Saturation : Saturate  UpperLimit=450  LowerLimit=-450  OutDataTypeMode=int16  OutDataType=fixdt(1, 16)  OutScaling=2^0  OutDataTypeStr=int16  RndMeth=Simplest
  Weighted Moving Average : simulink_need_slupdate/Weighted Moving Average  mgainval=[.1 .1 .1 .1 .1 .1 .1 .1 .1 .1]  vinit=0.0  samptime=-1  OutDataTypeStr=Inherit: Inherit via back propagation  OutDataType=sfix(16)  OutScaling=2^-10  DoSatur=off  GainDataType=uint(16)  MatRadixGroup=Best Precision: Matrix-wise  GainScaling=2^-10
  Out1 : Outport  OutDataType=fixdt(1, 16)  OutScaling=2^0  InitialOutput=50
  wires:
  Constant1/1 -> Map into range/5(out_max)
  Constant/1 -> Map into range/4(out_min)
  Demux/1 -> Map into range/2(in_min)
  Demux/2 -> Map into range/3(in_max)
  range/1 -> Data Type Conversion1/1
  Map into range/1(mappedValue) -> Saturation/1
  Data Type Conversion/1 -> Map into range/1(val)
  Data Type Conversion1/1 -> Demux/1
  input/1 -> Data Type Conversion/1
  Add 8% center deadband/1(Out1) -> Weighted Moving Average/1
  Saturation/1 -> Add 8% center deadband/1(In1)
  Gain/1 -> Out1/1
  Data Type Conversion2/1 -> Gain/1
  Weighted Moving Average/1 -> Data Type Conversion2/1

== system code_gen_HeadingHold/Controller/Radio Control Inputs1/If Action Subsystem2 ==
  Action Port : ActionPort  ActionType=then
  Constant : Constant  Value=0  OutDataType=fixdt(1, 16)  OutScaling=2^0  OutDataTypeStr=Inherit: Inherit via back propagation
  Out1 : Outport  OutDataType=fixdt(1, 16)  OutScaling=2^0  InitialOutput=0
  wires:
  Constant/1 -> Out1/1

== system code_gen_HeadingHold/Controller/Radio Control Inputs1/If Action Subsystem3 ==
  input : Inport  OutDataType=fixdt(1, 16)  OutScaling=2^0
  range : Inport  Port=2  OutDataType=fixdt(1, 16)  OutScaling=2^0
  Action Port : ActionPort  ActionType=else
  Add 5% deadband about 0 : Subsystem
  Constant : Constant  Value=-700  OutDataType=fixdt(1, 16)  OutScaling=2^0  OutDataTypeStr=Inherit: Inherit via back propagation
  Constant1 : Constant  Value=1000  OutDataType=fixdt(1, 16)  OutScaling=2^0  OutDataTypeStr=Inherit: Inherit via back propagation
  Data Type Conversion : DataTypeConversion  OutDataType=fixdt(1, 16)  OutScaling=2^0
  Data Type Conversion1 : DataTypeConversion  OutDataType=fixdt(1, 16)  OutScaling=2^0
  Demux : Demux  Outputs=2
  Map into range : Stateflow chart  TreatAsAtomicUnit=on
  Saturation : Saturate  UpperLimit=1000  LowerLimit=-700  OutDataTypeMode=int16  OutDataType=fixdt(1, 16)  OutScaling=2^0  OutDataTypeStr=int16  RndMeth=Simplest
  Out1 : Outport  OutDataType=fixdt(1, 16)  OutScaling=2^0  InitialOutput=0
  wires:
  Constant1/1 -> Map into range/5(out_max)
  Constant/1 -> Map into range/4(out_min)
  Demux/1 -> Map into range/2(in_min)
  Demux/2 -> Map into range/3(in_max)
  range/1 -> Data Type Conversion1/1
  Map into range/1(mappedValue) -> Saturation/1
  Data Type Conversion/1 -> Map into range/1(val)
  Data Type Conversion1/1 -> Demux/1
  Saturation/1 -> Add 5% deadband about 0/1(In1)
  input/1 -> Data Type Conversion/1
  Add 5% deadband about 0/1(Out1) -> Out1/1

== system code_gen_HeadingHold/Controller/Radio Control Inputs1/If Action Subsystem4 ==
  Action Port : ActionPort  ActionType=then
  Constant : Constant  Value=500  OutDataType=fixdt(1, 16)  OutScaling=2^0  OutDataTypeStr=Inherit: Inherit via back propagation
  Out1 : Outport  OutDataType=fixdt(1, 16)  OutScaling=2^0  InitialOutput=50
  wires:
  Constant/1 -> Out1/1
